simulink model "DirctSwork"  (Simulink 8.3)
settings: Solver=ode45  StartTime=0.0  StopTime=10.0  RelTol=1e-3
libraries: powerlib x4
settings Model: Creator=Administrator  LastModifiedBy=Administrator
settings DataIOCC: SignalLoggingSaveFormat=Dataset  InspectSignalLogs=on
settings DebuggingCC: UnderspecifiedInitializationDetection=Simplified  StateNameClashWarn=none
settings GRTTargetCC: CombineOutputUpdateFcns=on  GRTInterface=off

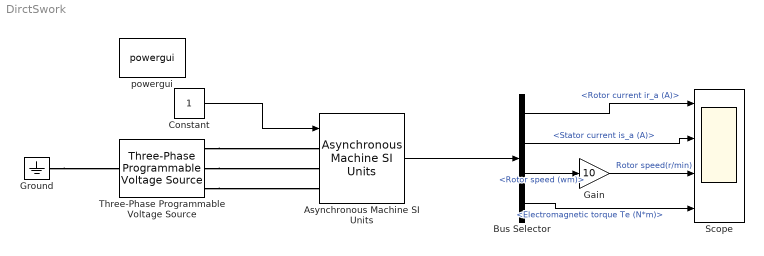
== system DirctSwork ==
  Asynchronous Machine SI Units : powerlib/Machines/Asynchronous Machine SI Units  PresetModel=No  MechanicalLoad=Torque Tm  ShowDetailedParameters=on  RotorType=Squirrel-cage  ReferenceFrame=Rotor  Units=SI  MeasurementBus=off  NominalParameters=[1500 380 50]  Stator=[0.435 0.002]  Rotor=[0.816 0.002]  Cage1=[ 0.022 0.226/377]  Cage2=[ 0.022 0.226/377]  Lm=0.6931  Mechanical=[0.089 0 2]  PolePairs=2  InitialConditions=[1 0 0 0 0 0 0 0]  SimulateSaturation=off  Saturation=[14.03593122, 27.81365428, 53.79336849, 72.68890987, 97.98006896, 148.6815601, 215.7428561, 302.9841135, 420.4778367 ; 230, 322, 414, 460, 506, 552, 598, 644, 690]  LoadFlowParameters=1492000  TsPowergui=0  TsBlock=-1  IterativeModel=Trapezoidal non iterative  Pmec=0
  Bus Selector : BusSelector  OutputSignals=Rotor measurements.Rotor current ir_a (A),Stator measurements.Stator current is_a (A),Mechanical.Rotor speed (wm),Mechanical.Electromagnetic torque Te (N*m)
  Constant : Constant  VectorParams1D=off
  Gain : Gain  Gain=10
  Ground : powerlib/Elements/Ground  LConnTagsString=a
  Scope : Scope  NumInputPorts=4
      settings: TickLabels=on  TimeRange=1  YMin=-5~-5~-5~-5  YMax=5~5~5~5
  Three-Phase Programmable Voltage Source : powerlib/Electrical Sources/Three-Phase Programmable Voltage Source  PositiveSequence=[268 0 50]  VariationEntity=None  VariationType=Table of time-amplitude pairs  VariationTypeAlt=Step  VariationStep=0.5  VariationRate=10  VariationMagnitude=0.3  VariationFrequency=2  VariationTiming=[1 2]  VariationPhaseA=off  Amplitudes=[1 0.8 1.2 1.0]  TimeValues=[0 0.1 0.15 0.2]  HarmonicGeneration=off  HarmonicA=[3 0.2 -25 0]  HarmonicB=[2 0.15 35 2]  Timing="[0.05  3]"  BusType=swing  Pref=0  Qref=0  Qmin=-inf  Qmax=inf
  powergui : powerlib/powergui  Priority=1  SimulationMode=Continuous  SolverType=Tustin  SampleTime=50e-6  frequency=60  SPID=off  DisableSnubberDevices=off  DisableRonSwitches=off  DisableVfSwitches=off  SwTol=0  Interpol=off  DisplayEquations=off  Ts=0  methode=off  frequencyindice=50  Pbase=100e6  ErrMax=1e-4  Iterations=50  UnitsV=kV  UnitsW=MW  FunctionMessages=off  echomessages=off  HookPort=off  EnableUseOfTLC=off  x0status=blocks  RestoreLinks=warning  ResistiveCurrentMeasurement=off  Frange=[0:2:500]  Ylog=off  Xlog=on  ShowGrid=off  save=off  variable=ZData  structure=0  ZoomFFT=off  StartTime=0.0  cycles=1  DisplayStyle=1  fundamental=60  FreqAxis=off  MaxFrequency=1000  frequencyindicesteady=1  RmsSteady=1  display=off
  wires:
  Constant/1 -> Asynchronous Machine SI Units/1
  Asynchronous Machine SI Units/1 -> Bus Selector/1
  Bus Selector/1 -> Scope/1  "<Rotor current ir_a (A)>"
  Bus Selector/2 -> Scope/2  "<Stator current is_a (A)>"
  Bus Selector/3 -> Gain/1  "<Rotor speed (wm)>"
  Gain/1 -> Scope/3  "Rotor speed(r/min)"
  Bus Selector/4 -> Scope/4  "<Electromagnetic torque Te (N*m)>"
  connections:
  Ground/LConn1 -- Three-Phase Programmable Voltage Source/LConn1
  Three-Phase Programmable Voltage Source/RConn1 -- Asynchronous Machine SI Units/LConn1
  Three-Phase Programmable Voltage Source/RConn2 -- Asynchronous Machine SI Units/LConn2
  Three-Phase Programmable Voltage Source/RConn3 -- Asynchronous Machine SI Units/LConn3
